simulink model "BANDARA_H_G_T_D_2022e048_Lab04_1"  (R2022b)
settings: Solver=VariableStepAuto  StartTime=0.0  StopTime=0.1  RelTol=1e-3
settings Model: Creator=DILANKA  LastModifiedBy=DILANKA

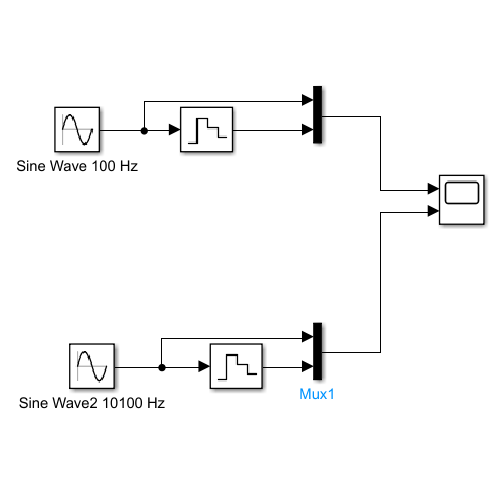
[thumbnail: Simulink's stored preview of the top-level diagram]
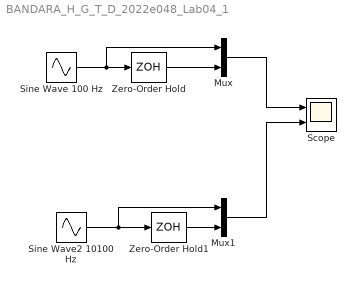
== system BANDARA_H_G_T_D_2022e048_Lab04_1 ==
  Mux : Mux  Inputs=2
  Mux1 : Mux  Inputs=2
  Scope : Scope  NumInputPorts=2
  Sine Wave 100 Hz : Sin  Frequency=100  SampleTime=0
  Sine Wave2 10100 Hz : Sin  Frequency=4000  SampleTime=0
  Zero-Order Hold : ZeroOrderHold  SampleTime=0.0001
  Zero-Order Hold1 : ZeroOrderHold  SampleTime=0.0001
  wires:
  Sine Wave2 10100 Hz/1 -> Mux1/1, Zero-Order Hold1/1
  Sine Wave 100 Hz/1 -> Mux/1, Zero-Order Hold/1
  Zero-Order Hold/1 -> Mux/2
  Mux/1 -> Scope/1
  Zero-Order Hold1/1 -> Mux1/2
  Mux1/1 -> Scope/2
